simulink model "AC_base_1_VSM_2_22a"  (R2022a)
settings: Solver=ode3  StartTime=0.0  StopTime=8  FixedStep=HWSampleTime  RelTol=1e-3
undefined symbols (not defined in the file): ControlSampleTime, DiscIntNeverNeededParam, HWSampleTime, Ipwm_back, Ipwm_off, LCL, Manage, Oversample, Param, scaling_factor, SM, Ts, V_DC, VSMCTRL
libraries: fl_lib x100, nesl_utility x63, simulink x38, FriedrichLibrary x38, ee_lib x20, simulink_extras x14, TriphaseHardwaremodule x12, spsEdgeDetectorLib x2, StateMachines x2, slpidlib x2, spsPower3phInstantaneousLib x1
(part 4 of 7)

== system AC_base_1_VSM_2_22a/Variant Subsystem3/VSM/VSM1/VSM/Meas ==
  note: Ucap reference frame
  note: VSM Reference Frame
  MEASIN : Inport
  "CONTROL " : Inport  Port=2
  Bus Creator : BusCreator  Inputs=4
  Bus Creator4 : BusCreator  Inputs=10
  Bus Selector : BusSelector  OutputSignals=meas_i_inverter,meas_u_cap,meas_u_out,meas_i_out,meas_vol_dc
  Bus Selector1 : BusSelector  OutputSignals=connection_state,enabled
  Bus Selector2 : BusSelector  OutputSignals=phi_VSM
  Gain{,1..3} (4 alike) : Gain  Gain=eye(3,NrChannels)  Multiplication=Matrix(K*u)
  InstantPowerPhN : FriedrichLibrary/Transformations/InstantPowerPhN  SystemSampleTime=-1  VariantActivationTime=update diagram  Latency=0  AutoFrameSizeCalculation=off
  "InstantPowerPhN " : FriedrichLibrary/Transformations/InstantPowerPhN  SystemSampleTime=-1  VariantActivationTime=update diagram  Latency=0  AutoFrameSizeCalculation=off
  PowerPu : Gain  Gain=2/3
  "PowerPu " : Gain  Gain=2/3
  "SI -> pu" : Subsystem  mask{PU=PU}
      mask prompts: PU "PU System"
      mask DialogControl ParameterGroupVar Prompt: Per Unit
  Signal Specification : SignalSpecification  Dimensions=1
  Signal Specification1 : SignalSpecification  Dimensions=1
  Signal Specification2 : SignalSpecification  Dimensions=3
  Signal Specification3 : SignalSpecification  Dimensions=1
  Symmetrical PLL : FriedrichLibrary/Discrete Stuff/Symmetrical PLL  Kp_PLL=PLL.kp  Ki_PLL=PLL.ki  Kd_PLL=0  Ts=ControlSampleTime
  f2omega : Gain  Gain=2*pi
  meas_i_inv : Subsystem
  meas_i_out : Subsystem
  meas_u_cap : Subsystem
  meas_u_out : Subsystem
  MEAS : Outport  VectorParamsAs1DForOutWhenUnconnected=off
  wires:
  PowerPu/1 -> Bus Creator4/8  "PQ"
  Gain3/1 -> meas_u_out/1(abc)
  meas_u_out/1(u_out_x) -> Bus Creator4/5  "u_out"
  Bus Selector/3 -> Gain3/1  "<meas_u_out>"
  Bus Creator/1 -> Bus Creator4/7  "PLL"
  Bus Selector/4 -> Gain2/1  "<meas_i_out>"
  Gain2/1 -> meas_i_out/1(abc), "InstantPowerPhN "/2
  meas_u_cap/1(u_cap_x) -> Bus Creator4/4  "u_cap"
  meas_i_inv/1(i_inv_x) -> Bus Creator4/3  "i_inv"
  InstantPowerPhN/1 -> PowerPu/1
  Bus Selector/2 -> Gain1/1  "<meas_u_cap>"
  Gain/1 -> InstantPowerPhN/2, meas_i_inv/1(abc)
  Symmetrical PLL/1 -> Signal Specification2/1  "vdq"
  Symmetrical PLL/3 -> Signal Specification/1  "f"
  Symmetrical PLL/2 -> Signal Specification1/1, meas_i_out/2(phi)  "phi"
  Bus Selector/1 -> Gain/1  "<meas_i_inverter>"
  Bus Selector/5 -> Signal Specification3/1  "<meas_vol_dc>"
  MEASIN/1 -> Bus Selector1/1, "SI -> pu"/1(MeasIn)
  "CONTROL "/1 -> Bus Selector2/1
  Signal Specification/1 -> f2omega/1, Bus Creator/3  "f"
  Signal Specification1/1 -> Bus Creator/2  "phi"
  Signal Specification2/1 -> Bus Creator/1  "vdq"
  f2omega/1 -> Bus Creator/4  "omega"
  "SI -> pu"/1(MeasOut) -> Bus Selector/1
  Signal Specification3/1 -> Bus Creator4/10  "u_dc"
  Bus Creator4/1 -> MEAS/1
  Bus Selector1/1 -> Bus Creator4/1  "<connection_state>"
  Bus Selector1/2 -> Bus Creator4/2  "<enabled>"
  Bus Selector2/1 -> meas_i_inv/2(phi), meas_u_out/2(phi), meas_u_cap/2(phi)  "<phi_VSM>"
  "InstantPowerPhN "/1 -> "PowerPu "/1
  "PowerPu "/1 -> Bus Creator4/9  "PQ_out"
  Gain1/1 -> meas_u_cap/1(abc), "InstantPowerPhN "/1, InstantPowerPhN/1, Symmetrical PLL/1
  meas_i_out/1(i_out_x) -> Bus Creator4/6  "i_out"

== system AC_base_1_VSM_2_22a/Variant Subsystem3/VSM/VSM1/command_center/Error ACK ==
  Toggle : Constant  OutMin=0  OutMax=1
  Out : Outport  VectorParamsAs1DForOutWhenUnconnected=off
  wires:
  Toggle/1 -> Out/1

== system AC_base_1_VSM_2_22a/Variant Subsystem3/VSM/VSM1/command_center/Shortcut1 ==

== system AC_base_1_VSM_2_22a/Variant Subsystem3/VSM/VSM1/command_center/Subsystem ==
  In1 : Inport
  In2 : Inport  Port=2
  Enable : EnablePort
  Constant : Constant  Value=4
  Display : Display
  TRI - WP : StateMachines/TRI - WP  Time_Pre1=0.1  T_Pre0=0.1  T_Connect=0.3  T_Disconnect=0.1  T_Enable=0.3  T_Disable=0.1  Time_Error=0.1  Ts=SM.TsTimer
  Terminator : Terminator
  Unit Delay : UnitDelay  SampleTime=ControlSampleTime  HasFrameUpgradeWarning=on
  Unit Delay1 : UnitDelay  SampleTime=ControlSampleTime  HasFrameUpgradeWarning=on
  precharge : Outport
  cmd_ac : Outport  Port=2
  wires:
  TRI - WP/3 -> cmd_ac/1
  In1/1 -> Unit Delay/1
  TRI - WP/4 -> Terminator/1
  Constant/1 -> TRI - WP/1
  Unit Delay1/1 -> TRI - WP/3
  Unit Delay/1 -> TRI - WP/2
  TRI - WP/1 -> Display/1
  TRI - WP/2 -> precharge/1  "precharge"
  In2/1 -> Unit Delay1/1

== system AC_base_1_VSM_2_22a/Variant Subsystem3/VSM/VSM1/command_center/cmd_VSM ==
  note: Parameter
  Bus Creator1 : BusCreator  Inputs=4
  Bus Creator2 : BusCreator  Inputs=2
  Current Control : Subsystem
  Damping : Subsystem
  Manage : Subsystem
  Virtual Circuit : Subsystem
  Virtual Synchronous Machine : Subsystem
  cmd_ac : Outport  VectorParamsAs1DForOutWhenUnconnected=off
  wires:
  Bus Creator2/1 -> cmd_ac/1
  Virtual Synchronous Machine/1(Virtual Synchronous Machine) -> Bus Creator1/1  "VSM"
  Current Control/1(Current Control) -> Bus Creator1/2  "CC"
  Damping/1(Damping) -> Bus Creator1/3  "Damping"
  Virtual Circuit/1(Virtual Circuit) -> Bus Creator1/4  "VC"
  Manage/1(Manage) -> Bus Creator2/1  "Manage"
  Bus Creator1/1 -> Bus Creator2/2  "Param"

== system AC_base_1_VSM_2_22a/Variant Subsystem3/VSM/VSM1/diagPlot/dq->abs1 ==
  dq : Inport
  Abs : Abs  SaturateOnIntegerOverflow=off
  Demux : Demux  Outputs=2
  Real-Imag to Complex : RealImagToComplex
  abs : Outport  VectorParamsAs1DForOutWhenUnconnected=off
  wires:
  Abs/1 -> abs/1
  Demux/2 -> Real-Imag to Complex/2
  dq/1 -> Demux/1
  Real-Imag to Complex/1 -> Abs/1
  Demux/1 -> Real-Imag to Complex/1

== system AC_base_1_VSM_2_22a/Variant Subsystem3/VSM/VSM1/diagPlot/dq0->abs ==
  dq0 : Inport
  Abs : Abs  SaturateOnIntegerOverflow=off
  Demux : Demux  Outputs=3
  Real-Imag to Complex : RealImagToComplex
  Terminator : Terminator
  abs : Outport  VectorParamsAs1DForOutWhenUnconnected=off
  wires:
  Demux/3 -> Terminator/1
  Demux/1 -> Real-Imag to Complex/1
  Real-Imag to Complex/1 -> Abs/1
  dq0/1 -> Demux/1
  Demux/2 -> Real-Imag to Complex/2
  Abs/1 -> abs/1

== system AC_base_1_VSM_2_22a/Variant Subsystem3/VSM/VSM1/diagPlot/dq0->abs2 ==
  dq0 : Inport
  Abs : Abs  SaturateOnIntegerOverflow=off
  Demux : Demux  Outputs=3
  Real-Imag to Complex : RealImagToComplex
  Terminator : Terminator
  abs : Outport  VectorParamsAs1DForOutWhenUnconnected=off
  wires:
  Demux/3 -> Terminator/1
  Demux/1 -> Real-Imag to Complex/1
  Real-Imag to Complex/1 -> Abs/1
  dq0/1 -> Demux/1
  Demux/2 -> Real-Imag to Complex/2
  Abs/1 -> abs/1

== system AC_base_1_VSM_2_22a/Variant Subsystem1/VSM/Inverter AverageMdl LC SimScape2/Modul F30 fixed DC voltage Average SimScape/measMerge3/measMerge123 ==
  note: In Triphase Modell: Mittelwert aus allen dc Spannungen.
      | Da im Modell die DC Spannung identisch ist, wird die erste übergeben
  meas1 : Inport
  meas2 : Inport  Port=2
  meas3 : Inport  Port=3
  Bus Creator : BusCreator  Inputs=3
  Bus Creator2 : BusCreator  Inputs=8
  Bus Selector : BusSelector  OutputSignals=meas1.meas_u_cap,meas2.meas_u_cap,meas3.meas_u_cap
  Bus Selector1 : BusSelector  OutputSignals=meas1.meas_u_out,meas2.meas_u_out,meas3.meas_u_out
  Bus Selector2 : BusSelector  OutputSignals=meas1.meas_i_inverter,meas2.meas_i_inverter,meas3.meas_i_inverter
  Bus Selector3 : BusSelector  OutputSignals=meas1.meas_i_out,meas2.meas_i_out,meas3.meas_i_out
  Bus Selector4 : BusSelector  OutputSignals=meas1.connection_state  OutputAsBus=on
  Bus Selector5 : BusSelector  OutputSignals=meas1.enabled  OutputAsBus=on
  Bus Selector6 : BusSelector  OutputSignals=meas1.meas_u_dc  OutputAsBus=on
  Bus Selector7 : BusSelector  OutputSignals=meas1.block,meas3.block,meas2.block
  Bus to Vector4 : BusToVector  Commented=on
  Mux{,1..4} (5 alike) : Mux  Inputs=3
  meas : Outport  VectorParamsAs1DForOutWhenUnconnected=off
  wires:
  Mux4/1 -> Bus Creator2/8  "block"
  Bus Selector7/3 -> Mux4/3  "<block>"
  Bus Selector7/1 -> Mux4/1  "<block>"
  Bus Selector7/2 -> Mux4/2  "<block>"
  Bus Selector3/3 -> Mux3/3  "<meas_i_out>"
  Bus Selector3/2 -> Mux3/2  "<meas_i_out>"
  Bus Selector3/1 -> Mux3/1  "<meas_i_out>"
  Bus Selector2/3 -> Mux2/3  "<meas_i_inverter>"
  Bus Selector2/2 -> Mux2/2  "<meas_i_inverter>"
  Bus Selector2/1 -> Mux2/1  "<meas_i_inverter>"
  Bus Selector1/3 -> Mux1/3  "<meas_u_out>"
  Bus Selector1/2 -> Mux1/2  "<meas_u_out>"
  Bus Selector1/1 -> Mux1/1  "<meas_u_out>"
  Bus Selector/3 -> Mux/3  "<meas_u_cap>"
  Bus Selector/2 -> Mux/2  "<meas_u_cap>"
  Bus Selector/1 -> Mux/1  "<meas_u_cap>"
  Bus Selector6/1 -> Bus Creator2/1  "meas_u_dc"
  Bus Selector5/1 -> Bus Creator2/7  "enabled"
  Bus Creator/1 -> Bus Selector6/1, Bus Selector/1, Bus Selector1/1, Bus Selector2/1, Bus Selector3/1, Bus Selector4/1, Bus Selector5/1, Bus Selector7/1
  meas2/1 -> Bus Creator/2  "meas2"
  meas1/1 -> Bus Creator/1  "meas1"
  Mux/1 -> Bus Creator2/2  "meas_u_cap"
  Mux1/1 -> Bus Creator2/3  "meas_u_out"
  Mux2/1 -> Bus Creator2/4  "meas_i_inverter"
  Mux3/1 -> Bus Creator2/5  "meas_i_out"
  Bus Creator2/1 -> meas/1
  Bus Selector4/1 -> Bus Creator2/6  "connection_state"
  meas3/1 -> Bus Creator/3  "meas3"

== system AC_base_1_VSM_2_22a/Variant Subsystem1/VSM/Inverter AverageMdl LC SimScape2/Modul F30 fixed DC voltage Average SimScape/simscape_bridgefilter_aca/PWM Blocking1 ==
  i_inverter : Inport
  enable : Inport  Port=2
  AND2 : Logic  IconShape=distinctive  AllPortsSameDT=off  OutDataTypeStr=boolean
  AND3 : Logic  IconShape=distinctive  AllPortsSameDT=off  OutDataTypeStr=boolean
  Abs2 : Abs  SaturateOnIntegerOverflow=off
  Compare To Constant1 : simulink/Logic and Bit Operations/Compare To Constant  relop=<=  const=Ipwm_back  OutDataTypeStr=boolean
  Compare To Constant4 : simulink/Logic and Bit Operations/Compare To Constant  relop=>  const=Ipwm_off  OutDataTypeStr=boolean
  Data Type Conversion2 : DataTypeConversion  SaturateOnIntegerOverflow=off  RndMeth=Floor
  S-R Flip-Flop1 : simulink_extras/Flip Flops/S-R Flip-Flop  initial_condition=0
  Terminator1 : Terminator
  Trigger Spike at new Control Sample : Subsystem
  Unit Delay2 : UnitDelay  SampleTime=-1  HasFrameUpgradeWarning=on
  enable_blk : Outport
  wires:
  i_inverter/1 -> Unit Delay2/1
  S-R Flip-Flop1/2 -> Terminator1/1
  AND3/1 -> Data Type Conversion2/1
  enable/1 -> AND3/1
  Data Type Conversion2/1 -> enable_blk/1
  S-R Flip-Flop1/1 -> AND3/2  "ena"
  Compare To Constant4/1 -> S-R Flip-Flop1/2  "R"
  AND2/1 -> S-R Flip-Flop1/1
  Abs2/1 -> Compare To Constant1/1, Compare To Constant4/1
  Unit Delay2/1 -> Abs2/1
  Compare To Constant1/1 -> AND2/2  "S"
  Trigger Spike at new Control Sample/1(y) -> AND2/1

== system AC_base_1_VSM_2_22a/Variant Subsystem1/VSM/Inverter AverageMdl LC SimScape2/Modul F30 fixed DC voltage Average SimScape/simscape_bridgefilter_aca1/PWM Blocking1 ==
  i_inverter : Inport
  enable : Inport  Port=2
  AND2 : Logic  IconShape=distinctive  AllPortsSameDT=off  OutDataTypeStr=boolean
  AND3 : Logic  IconShape=distinctive  AllPortsSameDT=off  OutDataTypeStr=boolean
  Abs2 : Abs  SaturateOnIntegerOverflow=off
  Compare To Constant1 : simulink/Logic and Bit Operations/Compare To Constant  relop=<=  const=Ipwm_back  OutDataTypeStr=boolean
  Compare To Constant4 : simulink/Logic and Bit Operations/Compare To Constant  relop=>  const=Ipwm_off  OutDataTypeStr=boolean
  Data Type Conversion2 : DataTypeConversion  SaturateOnIntegerOverflow=off  RndMeth=Floor
  S-R Flip-Flop1 : simulink_extras/Flip Flops/S-R Flip-Flop  initial_condition=0
  Terminator1 : Terminator
  Trigger Spike at new Control Sample : Subsystem
  Unit Delay2 : UnitDelay  SampleTime=-1  HasFrameUpgradeWarning=on
  enable_blk : Outport
  wires:
  Trigger Spike at new Control Sample/1(y) -> AND2/1
  Compare To Constant1/1 -> AND2/2  "S"
  Unit Delay2/1 -> Abs2/1
  Abs2/1 -> Compare To Constant4/1, Compare To Constant1/1
  AND2/1 -> S-R Flip-Flop1/1
  Compare To Constant4/1 -> S-R Flip-Flop1/2  "R"
  S-R Flip-Flop1/1 -> AND3/2  "ena"
  Data Type Conversion2/1 -> enable_blk/1
  enable/1 -> AND3/1
  AND3/1 -> Data Type Conversion2/1
  S-R Flip-Flop1/2 -> Terminator1/1
  i_inverter/1 -> Unit Delay2/1

== system AC_base_1_VSM_2_22a/Variant Subsystem1/VSM/Inverter AverageMdl LC SimScape2/Modul F30 fixed DC voltage Average SimScape/simscape_bridgefilter_aca2/PWM Blocking1 ==
  i_inverter : Inport
  enable : Inport  Port=2
  AND2 : Logic  IconShape=distinctive  AllPortsSameDT=off  OutDataTypeStr=boolean
  AND3 : Logic  IconShape=distinctive  AllPortsSameDT=off  OutDataTypeStr=boolean
  Abs2 : Abs  SaturateOnIntegerOverflow=off
  Compare To Constant1 : simulink/Logic and Bit Operations/Compare To Constant  relop=<=  const=Ipwm_back  OutDataTypeStr=boolean
  Compare To Constant4 : simulink/Logic and Bit Operations/Compare To Constant  relop=>  const=Ipwm_off  OutDataTypeStr=boolean
  Data Type Conversion2 : DataTypeConversion  SaturateOnIntegerOverflow=off  RndMeth=Floor
  S-R Flip-Flop1 : simulink_extras/Flip Flops/S-R Flip-Flop  initial_condition=0
  Terminator1 : Terminator
  Trigger Spike at new Control Sample : Subsystem
  Unit Delay2 : UnitDelay  SampleTime=-1  HasFrameUpgradeWarning=on
  enable_blk : Outport
  wires:
  i_inverter/1 -> Unit Delay2/1
  S-R Flip-Flop1/2 -> Terminator1/1
  AND3/1 -> Data Type Conversion2/1
  enable/1 -> AND3/1
  Data Type Conversion2/1 -> enable_blk/1
  S-R Flip-Flop1/1 -> AND3/2  "ena"
  Compare To Constant4/1 -> S-R Flip-Flop1/2  "R"
  AND2/1 -> S-R Flip-Flop1/1
  Abs2/1 -> Compare To Constant1/1, Compare To Constant4/1
  Unit Delay2/1 -> Abs2/1
  Compare To Constant1/1 -> AND2/2  "S"
  Trigger Spike at new Control Sample/1(y) -> AND2/1

== system AC_base_1_VSM_2_22a/Variant Subsystem1/VSM/VSM1/VSM/CONTROL/Subsystem1 ==
  <R1> : Inport
  <L1> : Inport  Port=2
  I : Inport  Port=3
  U_i : Inport  Port=4
  Enable : EnablePort
  MATLAB Function : MATLAB Function  TreatAsAtomicUnit=on  SystemSampleTime=ControlSampleTime
  Selector : Selector  InputPortWidth=3  IndexOptions=Index vector (dialog)  Indices=[1 2]  OutputSizes=1
  Selector1 : Selector  InputPortWidth=3  IndexOptions=Index vector (dialog)  Indices=[1 2]  OutputSizes=1
  phi_vsm : Outport
  U_v : Outport  Port=2
  wires:
  <L1>/1 -> MATLAB Function/2(L1)
  <R1>/1 -> MATLAB Function/3(R1)
  Selector/1 -> MATLAB Function/1(I)
  Selector1/1 -> MATLAB Function/4(U_i)
  I/1 -> Selector/1
  U_i/1 -> Selector1/1
  MATLAB Function/1(phi_vsm) -> phi_vsm/1
  MATLAB Function/2(U_v) -> U_v/1

== system AC_base_1_VSM_2_22a/Variant Subsystem1/VSM/VSM1/VSM/CONTROL/VSMOC1 ==
  Manage : Inport
  Meas : Inport  Port=2
  u_inv_dq : Inport  Port=3
  Bus Selector1 : BusSelector  OutputSignals=enable_VSM.enable_ctrl,Param.VSM,enable_VSM.enable_inertia,sp_VSM
  Bus Selector11 : BusSelector  OutputSignals=phi
  Bus Selector2 : BusSelector  OutputSignals=PQ,PLL,u_cap.u_cap_dq0
  Selector : Selector  InputPortWidth=3  IndexOptions=Index vector (dialog)  Indices=[1 2]  OutputSizes=1
  Switch : Switch  Criteria=u2 ~= 0  SaturateOnIntegerOverflow=off  InputSameDT=off
  VSMOC : Subsystem
  phi_rad : Outport  VectorParamsAs1DForOutWhenUnconnected=off
  sp_u_inv_dq : Outport  Port=2  InitialOutput=[1 0]  VectorParamsAs1DForOutWhenUnconnected=off
  VSMdiag : Outport  Port=3  VectorParamsAs1DForOutWhenUnconnected=off
  wires:
  Bus Selector2/1 -> VSMOC/4(PQ_meas)  "<PQ>"
  Selector/1 -> VSMOC/7(u_cap_dq1)
  Bus Selector2/3 -> Selector/1  "<u_cap_dq0>"
  u_inv_dq/1 -> VSMOC/6(u_inv_dq)
  Bus Selector1/4 -> VSMOC/3(sp_VSM)  "<sp_VSM>"
  Bus Selector1/3 -> VSMOC/2(enable_inertia)  "<enable_inertia>"
  Bus Selector1/2 -> VSMOC/1(Param)  "<VSM>"
  Bus Selector2/2 -> Bus Selector11/1, VSMOC/5(PLL)  "<PLL>"
  Meas/1 -> Bus Selector2/1
  Bus Selector1/1 -> Switch/2, VSMOC/Enable  "<enable_ctrl>"
  Manage/1 -> Bus Selector1/1
  Switch/1 -> phi_rad/1
  VSMOC/2(sp_u_inv_dq) -> sp_u_inv_dq/1
  VSMOC/3(VSMdiag) -> VSMdiag/1
  VSMOC/1(phi_rad) -> Switch/1
  Bus Selector11/1 -> Switch/3  "<phi>"

== system AC_base_1_VSM_2_22a/Variant Subsystem1/VSM/VSM1/VSM/CONTROL/Virtual Circuit mit R und L ==
  Param : Inport
  Reset : Inport  Port=2
  i_dq0 : Inport  Port=3
  Phi : Inport  Port=4
  Bus Selector : BusSelector  OutputSignals=R1,L1
  Bus Selector1 : BusSelector  OutputSignals=R1t,tauR,L1t,tauL
  Current Predictor : Subsystem  Commented=on
  L_Matrix : Gain  Gain=[0 -1 0;1 0 0; 0 0 0]
  L_Matrix1 : Gain  Gain=[0 -1 0;1 0 0; 0 0 0]
  PT1 : Subsystem  mask{K=1, Init=0, Ts=ControlSampleTime}
      mask prompts: K "Gain"; Init "Initial input"; Ts "Sample time"
      mask DialogControl DescGroupVar Prompt: PT1 discrete
      mask DialogControl DescTextVar Prompt: Simple discrete PT1
      mask Display:
      | text(0.5,0.5,get_param(gcb,'K'),'HorizontalAlignment','center','VerticalAlignment','Bottom')
      | text(0.5,0.5,'1 + s.tau','HorizontalAlignment','center','VerticalAlignment','Top')
      | plot([0.3 0.7],[0.5 0.5])
  PT2 : Subsystem  mask{K=1, Init=0, Ts=ControlSampleTime}
      mask prompts: K "Gain"; Init "Initial input"; Ts "Sample time"
      mask DialogControl DescGroupVar Prompt: PT1 discrete
      mask DialogControl DescTextVar Prompt: Simple discrete PT1
      mask Display:
      | text(0.5,0.5,get_param(gcb,'K'),'HorizontalAlignment','center','VerticalAlignment','Bottom')
      | text(0.5,0.5,'1 + s.tau','HorizontalAlignment','center','VerticalAlignment','Top')
      | plot([0.3 0.7],[0.5 0.5])
  "Param " : InportShadow
  Phi1 : InportShadow  Port=4
  Product : Product  Multiplication=Matrix(*)
  Product1 : Product  Multiplication=Matrix(*)
  Product2 : Product  Multiplication=Matrix(*)
  R_Matrix : Gain  Gain=[1 0 0;0 1 0; 0 0 0]
  R_Matrix1 : Gain  Gain=[1 0 0;0 1 0; 0 0 0]
  Reset1 : InportShadow  Port=2
  Sum : Sum  Inputs=++|
  Sum1 : Sum  Inputs=++|
  Sum2 : Sum  Inputs=|++
  " u_dq0" : Outport
  wires:
  Product/1 -> Sum2/1
  PT2/1(Y) -> Product2/2
  Reset1/1 -> PT2/3(Reset)
  Reset/1 -> PT1/3(Reset)
  Phi1/1 -> PT2/4(Phi)
  Phi/1 -> PT1/4(Phi)
  PT1/1(Y) -> Product1/2
  Sum2/1 -> " u_dq0"/1
  Product2/1 -> Sum1/2
  L_Matrix1/1 -> Product2/1
  Bus Selector1/3 -> L_Matrix1/1  "<L1t>"
  Bus Selector1/2 -> PT1/2(tau)  "<tauR>"
  Bus Selector1/4 -> PT2/2(tau)  "<tauL>"
  Bus Selector1/1 -> R_Matrix1/1  "<R1t>"
  Product1/1 -> Sum1/1
  R_Matrix1/1 -> Product1/1
  "Param "/1 -> Bus Selector1/1
  Sum/1 -> Product/1
  R_Matrix/1 -> Sum/2
  L_Matrix/1 -> Sum/1
  Bus Selector/2 -> L_Matrix/1  "<L1>"
  i_dq0/1 -> PT1/1(U), PT2/1(U), Product/2
  Bus Selector/1 -> R_Matrix/1  "<R1>"
  Param/1 -> Bus Selector/1

== system AC_base_1_VSM_2_22a/Variant Subsystem1/VSM/VSM1/VSM/CONTROL/Virtual Circuit1 ==
  Param : Inport
  Reset : Inport  Port=2
  i_dq0 : Inport  Port=3
  Phi : Inport  Port=4
  Bus Selector : BusSelector  OutputSignals=R1,L1
  Bus Selector1 : BusSelector  OutputSignals=R1t,tauR,L1t,tauL
  Current Predictor : Subsystem  Commented=on
  L_Matrix : Gain  Gain=[0 -1 0;1 0 0; 0 0 0]
  L_Matrix1 : Gain  Gain=[0 -1 0;1 0 0; 0 0 0]
  PT1 : Subsystem  mask{K=1, Init=0, Ts=ControlSampleTime}
      mask prompts: K "Gain"; Init "Initial input"; Ts "Sample time"
      mask DialogControl DescGroupVar Prompt: PT1 discrete
      mask DialogControl DescTextVar Prompt: Simple discrete PT1
      mask Display:
      | text(0.5,0.5,get_param(gcb,'K'),'HorizontalAlignment','center','VerticalAlignment','Bottom')
      | text(0.5,0.5,'1 + s.tau','HorizontalAlignment','center','VerticalAlignment','Top')
      | plot([0.3 0.7],[0.5 0.5])
  PT2 : Subsystem  Commented=on  mask{K=1, Init=0, Ts=ControlSampleTime}
      mask prompts: K "Gain"; Init "Initial input"; Ts "Sample time"
      mask DialogControl DescGroupVar Prompt: PT1 discrete
      mask DialogControl DescTextVar Prompt: Simple discrete PT1
      mask Display:
      | text(0.5,0.5,get_param(gcb,'K'),'HorizontalAlignment','center','VerticalAlignment','Bottom')
      | text(0.5,0.5,'1 + s.tau','HorizontalAlignment','center','VerticalAlignment','Top')
      | plot([0.3 0.7],[0.5 0.5])
  "Param " : InportShadow
  Phi1 : InportShadow  Port=4
  Product : Product  Multiplication=Matrix(*)
  Product1 : Product  Multiplication=Matrix(*)
  Product2 : Product  Commented=on  Multiplication=Matrix(*)
  Product3 : Product  Multiplication=Matrix(*)
  R_Matrix : Gain  Gain=[1 0 0;0 1 0; 0 0 0]
  R_Matrix1 : Gain  Gain=[1 0 0;0 1 0; 0 0 0]
  Reset1 : InportShadow  Port=2
  Scope : Scope  NumInputPorts=2
  Scope1 : Scope
  Sum : Sum  Inputs=++|
  Sum1 : Sum  Inputs=++|
  Sum2 : Sum  Inputs=|++
  " u_dq0" : Outport
  wires:
  Product3/1 -> Scope/1
  Reset1/1 -> PT2/3(Reset)
  Reset/1 -> PT1/3(Reset)
  Phi1/1 -> PT2/4(Phi)
  PT1/1(Y) -> Product1/2
  Sum2/1 -> " u_dq0"/1
  Sum1/1 -> Sum2/2
  Product2/1 -> Sum1/2, Scope1/1
  PT2/1(Y) -> Product2/2
  L_Matrix1/1 -> Product2/1
  Bus Selector1/3 -> L_Matrix1/1  "<L1t>"
  Bus Selector1/2 -> PT1/2(tau)  "<tauR>"
  Bus Selector1/4 -> PT2/2(tau)  "<tauL>"
  Bus Selector1/1 -> R_Matrix1/1  "<R1t>"
  Product1/1 -> Sum1/1, Scope/2
  R_Matrix1/1 -> Product1/1
  Product/1 -> Sum2/1
  "Param "/1 -> Bus Selector1/1
  Sum/1 -> Product/1
  R_Matrix/1 -> Sum/2, Product3/1
  L_Matrix/1 -> Sum/1
  Bus Selector/2 -> L_Matrix/1  "<L1>"
  i_dq0/1 -> Product/2, Product3/2, PT1/1(U), PT2/1(U)
  Bus Selector/1 -> R_Matrix/1  "<R1>"
  Param/1 -> Bus Selector/1

== system AC_base_1_VSM_2_22a/Variant Subsystem1/VSM/VSM1/VSM/CONTROL/active_damping ==
  enable_damp_dq : Inport
  Reset : Inport  Port=2
  u_dq0 : Inport  Port=3
  Phi : Inport  Port=4
  Bus Selector : BusSelector  OutputSignals=Damp_dq,Damp_dq,Damp_CM,OmLead,OmLag
  Integrator (inertia) : DiscreteIntegrator  gainval=1  ExternalReset=rising  InitialConditionSource=external  InitialCondition=1  SampleTime=ControlSampleTime  ICPrevOutput=DiscIntNeverNeededParam  ICPrevScaledInput=DiscIntNeverNeededParam
  Mux : Mux  Inputs=3
  Product{,1..3} (4 alike) : Product
  Sum : Sum  Inputs=|+-
  Sum2 : Sum  Inputs=++|
  Unit Delay2 : UnitDelay  InitialCondition=[0 0 0]  SampleTime=ControlSampleTime  HasFrameUpgradeWarning=on
  dq0->ab0 phi : FriedrichLibrary/Transformations/dq0->ab0 phi  SystemSampleTime=-1  VariantActivationTime=update diagram  Latency=0  AutoFrameSizeCalculation=off
  damp_dq0 : Outport  VectorParamsAs1DForOutWhenUnconnected=off
  wires:
  Bus Selector/5 -> Product3/2  "<OmLag>"
  Bus Selector/4 -> Product2/1  "<OmLead>"
  dq0->ab0 phi/1 -> Integrator (inertia)/3
  Unit Delay2/1 -> dq0->ab0 phi/1
  Reset/1 -> Integrator (inertia)/2
  Phi/1 -> dq0->ab0 phi/2
  Product1/1 -> damp_dq0/1
  Mux/1 -> Product/1, Product1/1  "enable"
  Product/1 -> Product2/2, Sum2/1
  u_dq0/1 -> Product/2
  Bus Selector/3 -> Mux/3  "<Damp_CM>"
  Bus Selector/2 -> Mux/2  "<Damp_dq>"
  Bus Selector/1 -> Mux/1  "<Damp_dq>"
  enable_damp_dq/1 -> Bus Selector/1
  Sum/1 -> Integrator (inertia)/1
  Sum2/1 -> Product1/2, Product3/1
  Product3/1 -> Sum/2
  Integrator (inertia)/1 -> Sum2/2, Unit Delay2/1
  Product2/1 -> Sum/1

== system AC_base_1_VSM_2_22a/Variant Subsystem1/VSM/VSM1/VSM/CONTROL/dq0 to duty ==
  phi_rad : Inport
  u_dq0 : Inport  Port=2
  u_dc : Inport  Port=3
  Bias : Bias  Bias=Ctrl.PWM.tauT*Ctrl.PU.omegab  SaturateOnIntegerOverflow=off
  Bus Creator3 : BusCreator  Inputs=2
  Divide : Product  Inputs=*/
  Gain : Gain  Gain=eye(NrChannels,3)  Multiplication=Matrix(K*u)
  Modulation : FriedrichLibrary/Transformations/Modulation  Method=Sine Modulation  Ts=ControlSampleTime
  SMA : FriedrichLibrary/Discrete Stuff/SMA  n_samples=1/ControlSampleTime/100  init_out=0
  Saturation : Saturate  UpperLimit=inf  LowerLimit=1
  Signal Specification1 : SignalSpecification
  dq0->ab0 phi : FriedrichLibrary/Transformations/dq0->ab0 phi  SystemSampleTime=-1  VariantActivationTime=update diagram  Latency=0  AutoFrameSizeCalculation=off
  d : Outport  VectorParamsAs1DForOutWhenUnconnected=off
  pwmDiag : Outport  Port=2  VectorParamsAs1DForOutWhenUnconnected=off
  wires:
  SMA/1 -> Divide/2
  Saturation/1 -> SMA/1
  Signal Specification1/1 -> d/1
  Gain/1 -> Signal Specification1/1, Bus Creator3/1  "pwm"
  Bus Creator3/1 -> pwmDiag/1  "pwmDiag"
  u_dc/1 -> Saturation/1
  Bias/1 -> dq0->ab0 phi/2
  Modulation/1 -> Gain/1
  dq0->ab0 phi/1 -> Divide/1
  Divide/1 -> Modulation/1  "ab0 norm"
  u_dq0/1 -> dq0->ab0 phi/1
  phi_rad/1 -> Bias/1, Bus Creator3/2  "phi"

== system AC_base_1_VSM_2_22a/Variant Subsystem1/VSM/VSM1/VSM/CONTROL/i_dq_ctrl ==
  note: PI Control
  note: Outrouting
  note: Inrouting
  Param : Inport
  enable_cc : Inport  Port=2
  sp_cc : Inport  Port=3
  ms_i_inv_dq : Inport  Port=4
  u_ff_dq : Inport  Port=5
  u_inv_dq : Inport  Port=6
  Enable : EnablePort  StatesWhenEnabling=reset
  Bus Creator2 : BusCreator  Inputs=4
  Bus Selector13 : BusSelector  OutputSignals=init_u_inv
  Constant : Constant
  Demux : Demux  Outputs=2
  From1 : From  Commented=on  GotoTag=initU
  Gain1 : Gain  Commented=on  Gain=Kff
  Gain2 : Gain  Gain=L_inv
  Gain4 : Gain  Gain=[0 -1;1 0]  Multiplication=Matrix(K*u)
  Gain5 : Gain  Commented=on  Gain=1-Kff
  Mux : Mux  Inputs=2
  PI : Subsystem
  Product : Product
  Product1 : Product
  Product2 : Product
  Scope : Scope  NumInputPorts=3
  Step : Step  Time=8  Before=1  After=0  SampleTime=0
  Sum1 : Sum  Inputs=+++
  Sum2 : Sum  Commented=on  Inputs=|+-
  Sum3 : Sum  Inputs=|+-
  Switch1 : Switch  Commented=on  Criteria=u2 > Threshold  SaturateOnIntegerOverflow=off  InputSameDT=off
  sp_u_inv_dq : Outport  VectorParamsAs1DForOutWhenUnconnected=off
  CCdiag : Outport  Port=2  VectorParamsAs1DForOutWhenUnconnected=off
  wires:
  PI/1(u) -> Sum1/1  "pi"
  Constant/1 -> Product1/2, Product2/2
  Demux/1 -> Product2/1
  Product2/1 -> Mux/1
  Product1/1 -> Mux/2
  Demux/2 -> Product1/1
  Mux/1 -> PI/1(di)
  ms_i_inv_dq/1 -> Gain4/1, Sum3/2, [i_dq]
  Product/1 -> [sp_u_dq], sp_u_inv_dq/1
  Gain5/1 -> Switch1/3
  u_ff_dq/1 -> Gain5/1, Gain1/1, PI/2(u0), Scope/2
  [i_dq] -> Bus Creator2/2  "i_dq"
  [sp_i_dq] -> Bus Creator2/1  "sp_i_dq"
  Bus Creator2/1 -> CCdiag/1
  [Enable] -> Bus Creator2/4  "enable_cc"
  enable_cc/1 -> [Enable]  "enable_cc"
  [sp_u_dq] -> Bus Creator2/3  "sp_u_dq"
  [Enable] -> Product/1
  Bus Selector13/1 -> [initU]  "<init_u_inv>"
  Param/1 -> Bus Selector13/1
  sp_cc/1 -> Sum3/1, [sp_i_dq]
  Sum3/1 -> Demux/1
  [Enable] -> PI/Enable
  u_inv_dq/1 -> Switch1/1
  Sum1/1 -> Product/2, Scope/1
  From1/1 -> Switch1/2
  Gain2/1 -> Sum2/2  "dq decouple"
  Gain4/1 -> Gain2/1
  Switch1/1 -> Sum2/1

== system AC_base_1_VSM_2_22a/Variant Subsystem1/VSM/VSM1/VSM/MANAGEMENT/Subsystem1 ==
  i_inv_ab : Inport
  <i_inv_dq0> : Inport  Port=2
  <u_cap_ab0> : Inport  Port=3
  <PQ_out> : Inport  Port=4
  enable : Inport  Port=5
  i_out_ab : Inport  Port=6
  "AL brechen AL nicht mit FCN lösbar " : Memory
  Compare To Constant : simulink/Logic and Bit Operations/Compare To Constant  relop===  const=0  OutDataTypeStr=boolean
  Complex to Magnitude-Angle : ComplexToMagnitudeAngle
  Demux : Demux  Outputs=2
  Divide : Product  Inputs=*/
  Enabled Subsystem : Subsystem  TreatAsAtomicUnit=on
  Math Function1 : Math  Operator=square  SignedPower=on
  Math Function2 : Math  Operator=square  SignedPower=on
  Math Function3 : Math  Operator=square  SignedPower=on
  Max : MinMax  Function=max  Inputs=2
  Real-Imag to Complex : RealImagToComplex
  Scope : Scope  NumInputPorts=2
  Selector2 : Selector  InputPortWidth=3  IndexOptions=Index vector (dialog)  Indices=[1 2]  OutputSizes=1
  Sqrt1 : Sqrt
  Sqrt2 : Sqrt
  Sqrt3 : Sqrt
  Subsystem : Subsystem
  Sum of Elements1 : Sum  Inputs=+
  Sum of Elements2 : Sum  Inputs=+
  Sum of Elements3 : Sum  Inputs=+
  Transport Delay : TransportDelay  DelayTime=0.1
  Transport Delay1 : TransportDelay  DelayTime=0.1
  Unit Delay : UnitDelay  SampleTime=ControlSampleTime  HasFrameUpgradeWarning=on
  Unit Delay1 : UnitDelay  SampleTime=ControlSampleTime  HasFrameUpgradeWarning=on
  CC : Outport
  sp_CC : Outport  Port=2
  wires:
  Complex to Magnitude-Angle/2 -> Subsystem/7(angle_i)
  Real-Imag to Complex/1 -> Complex to Magnitude-Angle/1
  Divide/1 -> Transport Delay1/1, Demux/1
  Demux/2 -> Real-Imag to Complex/2
  Demux/1 -> Real-Imag to Complex/1
  Max/1 -> Subsystem/3(iabs)
  Sqrt2/1 -> Transport Delay/1, Max/2
  Sqrt3/1 -> Max/1
  i_out_ab/1 -> Math Function3/1
  Sum of Elements3/1 -> Sqrt3/1
  Math Function3/1 -> Sum of Elements3/1
  Transport Delay1/1 -> Enabled Subsystem/2(i_pq)
  Unit Delay1/1 -> Subsystem/5(PQ_pre)
  Enabled Subsystem/2(i_pq_pre) -> Scope/2, Unit Delay1/1
  Unit Delay/1 -> Subsystem/6(i abs_pre)
  Transport Delay/1 -> Enabled Subsystem/1(i_abs)
  Subsystem/3(set) -> Compare To Constant/1
  Enabled Subsystem/1(i abs_pre) -> Unit Delay/1, Scope/1
  Compare To Constant/1 -> Enabled Subsystem/Enable
  enable/1 -> Subsystem/Enable
  <PQ_out>/1 -> Subsystem/2(PQ_out), Divide/1
  Subsystem/2(CC) -> CC/1
  i_inv_ab/1 -> Math Function1/1
  Subsystem/1(i_sp) -> sp_CC/1  "sp_CC"
  <i_inv_dq0>/1 -> "AL brechen AL nicht mit FCN lösbar "/1
  <u_cap_ab0>/1 -> Selector2/1
  Math Function2/1 -> Sum of Elements2/1
  Sqrt1/1 -> Divide/2, Subsystem/4(U_cap)
  "AL brechen AL nicht mit FCN lösbar "/1 -> Subsystem/1(i_inv)
  Sum of Elements2/1 -> Sqrt1/1
  Math Function1/1 -> Sum of Elements1/1
  Selector2/1 -> Math Function2/1
  Sum of Elements1/1 -> Sqrt2/1

== system AC_base_1_VSM_2_22a/Variant Subsystem1/VSM/VSM1/VSM/MANAGEMENT/current_watchdog ==
  |i| set : Inport
  |i| reset : Inport  Port=2
  i_ab : Inport  Port=3
  sp_gain : Inport  Port=4
  PQ : Inport  Port=5
  i_inv : Inport  Port=6
  active_current_watchdog : EnablePort  StatesWhenEnabling=reset
  Divide : Product  Inputs=/**
  MATLAB Function : MATLAB Function  Commented=on  TreatAsAtomicUnit=on
  Math Function1 : Math  Operator=square  SignedPower=on
  Math Function2 : Math  Operator=square  SignedPower=on
  Math Function3 : Math  Operator=square  SignedPower=on
  Relational Operator : RelationalOperator  Operator=<=  OutDataTypeStr=boolean  InputSameDT=off
  Relational Operator1 : RelationalOperator  Operator=<=  OutDataTypeStr=boolean  InputSameDT=off
  S-R Flip-Flop1 : simulink_extras/Flip Flops/S-R Flip-Flop  initial_condition=0
  Scope : Scope  NumInputPorts=3
  Scope1 : Scope
  Sum of Elements1 : Sum  Inputs=+
  Terminator1 : Terminator
  enable_cc : Outport  VectorParamsAs1DForOutWhenUnconnected=off
  sp_gain_wd : Outport  Port=2  VectorParamsAs1DForOutWhenUnconnected=off
  wires:
  i_inv/1 -> MATLAB Function/4(i_inv)
  PQ/1 -> MATLAB Function/3(p), Scope1/1
  MATLAB Function/2(i) -> sp_gain_wd/1
  MATLAB Function/1(CC) -> Scope/1, enable_cc/1
  sp_gain/1 -> Divide/3
  |i| set/1 -> Math Function2/1, Divide/1
  |i| reset/1 -> Math Function3/1, Divide/2
  Math Function3/1 -> Relational Operator1/2
  S-R Flip-Flop1/2 -> Terminator1/1
  Relational Operator1/1 -> S-R Flip-Flop1/2
  Math Function1/1 -> Sum of Elements1/1
  Sum of Elements1/1 -> Relational Operator/2, MATLAB Function/1(abs), Relational Operator1/1
  i_ab/1 -> Math Function1/1
  Math Function2/1 -> MATLAB Function/2(set), Relational Operator/1

== system AC_base_1_VSM_2_22a/Variant Subsystem1/VSM/VSM1/VSM/MANAGEMENT/sp_VSM ==
  EnableRateLimit : Inport
  CMD : Inport  Port=2
  MEAS : Inport  Port=3
  Bus Creator : BusCreator  Inputs=3
  Bus Selector1 : BusSelector  OutputSignals=u_out.u_out_ab0
  Bus Selector6 : BusSelector  OutputSignals=Param.VSM.sp_f,Param.VSM.sp_E,Param.VSM.sp_PQ,Param.VSM.sp_PQ_limit
  "CMD " : InportShadow  Port=2
  E(PQ) : Subsystem
  PQ(U) Limit : Subsystem
  RateLimit : Subsystem
  Saturation : Saturate  UpperLimit=1  LowerLimit=-1
  sp_VSM : Outport  VectorParamsAs1DForOutWhenUnconnected=off
  wires:
  Saturation/1 -> RateLimit/1(PQ)
  "CMD "/1 -> E(PQ)/2(cmd)
  Bus Creator/1 -> sp_VSM/1
  Bus Selector6/1 -> Bus Creator/1  "<sp_f>"
  MEAS/1 -> Bus Selector1/1
  CMD/1 -> Bus Selector6/1
  PQ(U) Limit/1(sp_PQ_limit) -> Bus Creator/3  "sp_PQ"
  Bus Selector6/4 -> PQ(U) Limit/2(enable)  "<sp_PQ_limit>"
  Bus Selector1/1 -> PQ(U) Limit/3(u_out)  "<u_out_ab0>"
  RateLimit/1(PQslow) -> PQ(U) Limit/1(sp_PQ), E(PQ)/3(sp_PQ)
  EnableRateLimit/1 -> RateLimit/Enable  "ENABLED"
  Bus Selector6/3 -> Saturation/1  "<sp_PQ>"
  Bus Selector6/2 -> E(PQ)/1(E)  "<sp_E>"
  E(PQ)/1(sp_E) -> Bus Creator/2  "sp_E"

== system AC_base_1_VSM_2_22a/Variant Subsystem1/VSM/VSM1/VSM/Meas/SI -> pu ==
  MeasIn : Inport
  Bus Creator1 : BusCreator  Inputs=5
  Bus Selector : BusSelector  OutputSignals=meas_u_out,meas_i_out,meas_i_inverter,meas_u_dc,meas_u_cap
  Normalize : Gain  Gain=1/PU.Ub  OutDataTypeStr=double  RndMeth=Round
  Normalize1 : Gain  Gain=1/PU.Ib  OutDataTypeStr=double  RndMeth=Round
  Normalize2 : Gain  Gain=1/PU.Ib  OutDataTypeStr=double  RndMeth=Round
  Normalize3 : Gain  Gain=1/PU.Ub  OutDataTypeStr=double  RndMeth=Round
  Normalize4 : Gain  Gain=1/PU.Ub/2  OutDataTypeStr=double  RndMeth=Round
  MeasOut : Outport  VectorParamsAs1DForOutWhenUnconnected=off
  wires:
  MeasIn/1 -> Bus Selector/1
  Normalize/1 -> Bus Creator1/1  "meas_u_out"
  Normalize1/1 -> Bus Creator1/3  "meas_i_inverter"
  Normalize2/1 -> Bus Creator1/2  "meas_i_out"
  Normalize4/1 -> Bus Creator1/4  "meas_vol_dc"
  Bus Creator1/1 -> MeasOut/1
  Bus Selector/1 -> Normalize/1  "<meas_u_out>"
  Bus Selector/2 -> Normalize2/1  "<meas_i_out>"
  Bus Selector/3 -> Normalize1/1  "<meas_i_inverter>"
  Bus Selector/4 -> Normalize4/1  "<meas_u_dc>"
  Bus Selector/5 -> Normalize3/1  "<meas_u_cap>"
  Normalize3/1 -> Bus Creator1/5  "meas_u_cap"

== system AC_base_1_VSM_2_22a/Variant Subsystem1/VSM/VSM1/VSM/Meas/meas_i_inv ==
  abc : Inport
  phi : Inport  Port=2
  Bus Creator1 : BusCreator  Inputs=3
  PhN->ab2 : FriedrichLibrary/Transformations/PhN->ab0  SystemSampleTime=-1  VariantActivationTime=update diagram  Latency=0  AutoFrameSizeCalculation=off
  ab0->dq0-faster : FriedrichLibrary/Transformations/ab0->dq0-faster  SystemSampleTime=-1  VariantActivationTime=update diagram  Latency=0  AutoFrameSizeCalculation=off
  i_inv_x : Outport  VectorParamsAs1DForOutWhenUnconnected=off
  wires:
  Bus Creator1/1 -> i_inv_x/1
  phi/1 -> ab0->dq0-faster/2
  abc/1 -> PhN->ab2/1, Bus Creator1/1  "i_inv_abc"
  PhN->ab2/1 -> ab0->dq0-faster/1, Bus Creator1/2  "i_inv_ab0"
  ab0->dq0-faster/1 -> Bus Creator1/3  "i_inv_dq0"

== system AC_base_1_VSM_2_22a/Variant Subsystem1/VSM/VSM1/VSM/Meas/meas_i_out ==
  abc : Inport
  phi : Inport  Port=2
  Bus Creator1 : BusCreator  Inputs=3
  PhN->ab2 : FriedrichLibrary/Transformations/PhN->ab0  SystemSampleTime=-1  VariantActivationTime=update diagram  Latency=0  AutoFrameSizeCalculation=off
  ab0->dq0-faster : FriedrichLibrary/Transformations/ab0->dq0-faster  SystemSampleTime=-1  VariantActivationTime=update diagram  Latency=0  AutoFrameSizeCalculation=off
  i_out_x : Outport  VectorParamsAs1DForOutWhenUnconnected=off
  wires:
  Bus Creator1/1 -> i_out_x/1
  phi/1 -> ab0->dq0-faster/2
  abc/1 -> PhN->ab2/1, Bus Creator1/1  "i_out_abc"
  PhN->ab2/1 -> ab0->dq0-faster/1, Bus Creator1/2  "i_out_ab0"
  ab0->dq0-faster/1 -> Bus Creator1/3  "i_out_dq0"

== system AC_base_1_VSM_2_22a/Variant Subsystem1/VSM/VSM1/VSM/Meas/meas_u_cap ==
  abc : Inport
  phi : Inport  Port=2
  Bus Creator1 : BusCreator  Inputs=3
  PhN->ab2 : FriedrichLibrary/Transformations/PhN->ab0  SystemSampleTime=-1  VariantActivationTime=update diagram  Latency=0  AutoFrameSizeCalculation=off
  ab0->dq0-faster : FriedrichLibrary/Transformations/ab0->dq0-faster  SystemSampleTime=-1  VariantActivationTime=update diagram  Latency=0  AutoFrameSizeCalculation=off
  u_cap_x : Outport  VectorParamsAs1DForOutWhenUnconnected=off
  wires:
  ab0->dq0-faster/1 -> Bus Creator1/3  "u_cap_dq0"
  PhN->ab2/1 -> Bus Creator1/2, ab0->dq0-faster/1  "u_cap_ab0"
  abc/1 -> Bus Creator1/1, PhN->ab2/1  "u_cap_abc"
  phi/1 -> ab0->dq0-faster/2
  Bus Creator1/1 -> u_cap_x/1

== system AC_base_1_VSM_2_22a/Variant Subsystem1/VSM/VSM1/VSM/Meas/meas_u_out ==
  abc : Inport
  phi : Inport  Port=2
  Bus Creator1 : BusCreator  Inputs=3
  PhN->ab2 : FriedrichLibrary/Transformations/PhN->ab0  SystemSampleTime=-1  VariantActivationTime=update diagram  Latency=0  AutoFrameSizeCalculation=off
  ab0->dq0-faster : FriedrichLibrary/Transformations/ab0->dq0-faster  SystemSampleTime=-1  VariantActivationTime=update diagram  Latency=0  AutoFrameSizeCalculation=off
  u_out_x : Outport  VectorParamsAs1DForOutWhenUnconnected=off
  wires:
  ab0->dq0-faster/1 -> Bus Creator1/3  "u_out_dq0"
  PhN->ab2/1 -> Bus Creator1/2, ab0->dq0-faster/1  "u_out_ab0"
  abc/1 -> Bus Creator1/1, PhN->ab2/1  "u_out_abc"
  phi/1 -> ab0->dq0-faster/2
  Bus Creator1/1 -> u_out_x/1

== system AC_base_1_VSM_2_22a/Variant Subsystem1/VSM/VSM1/command_center/cmd_VSM/Current Control ==
  note: else: init with u cap
  Bus Creator6 : BusCreator  Inputs=5
  Bus Creator7 : BusCreator  Inputs=3
  Init with u_inv [0/1] : Constant  Value=VSMCTRL.CC.init_uinv
  activate : Constant  Value=VSMCTRL.CC.activate
  external_stop_cc1 : Constant  Value=0
  external_stop_cc4 : Constant  Value=0
  i_reset_abs : Constant  Value=VSMCTRL.CC.i_reset
  i_set_abs : Constant  Value=VSMCTRL.CC.i_set
  i_sp_gain : Constant  Value=VSMCTRL.CC.i_sp_gain
  Current Control : Outport  VectorParamsAs1DForOutWhenUnconnected=off
  wires:
  Bus Creator6/1 -> Current Control/1  "CC"
  Init with u_inv [0/1]/1 -> Bus Creator6/1  "init_u_inv"
  external_stop_cc1/1 -> Bus Creator6/3  "ex_stop_cc"
  i_sp_gain/1 -> Bus Creator6/4  "i_sp_gain"
  i_set_abs/1 -> Bus Creator7/2  "abs_i_set"
  external_stop_cc4/1 -> Bus Creator6/2  "ex_start_cc"
  Bus Creator7/1 -> Bus Creator6/5  "watchdog"
  i_reset_abs/1 -> Bus Creator7/3  "abs_i_reset"
  activate/1 -> Bus Creator7/1  "activate"

== system AC_base_1_VSM_2_22a/Variant Subsystem1/VSM/VSM1/command_center/cmd_VSM/Damping ==
  Bus Creator5 : BusCreator  Inputs=4
  EnableDamp_CM [0/1] : Constant  Value=VSMCTRL.VTFF.EnableCM
  EnableDamp_dq [0/1] : Constant  Value=VSMCTRL.VTFF.EnableDQ
  Omega Lag : Constant  Value=VSMCTRL.VTFF.OmLag
  Omega Lead : Constant  Value=VSMCTRL.VTFF.OmLead
  Damping : Outport  VectorParamsAs1DForOutWhenUnconnected=off
  wires:
  Omega Lag/1 -> Bus Creator5/4  "OmLag"
  Omega Lead/1 -> Bus Creator5/3  "OmLead"
  Bus Creator5/1 -> Damping/1
  EnableDamp_dq [0/1]/1 -> Bus Creator5/1  "Damp_dq"
  EnableDamp_CM [0/1]/1 -> Bus Creator5/2  "Damp_CM"

== system AC_base_1_VSM_2_22a/Variant Subsystem1/VSM/VSM1/command_center/cmd_VSM/Manage ==
  Bus Creator : BusCreator  Inputs=2
  connect : Constant
  enable : Constant
  Manage : Outport  VectorParamsAs1DForOutWhenUnconnected=off
  wires:
  enable/1 -> Bus Creator/2  "enable"
  connect/1 -> Bus Creator/1  "connect"
  Bus Creator/1 -> Manage/1

== system AC_base_1_VSM_2_22a/Variant Subsystem1/VSM/VSM1/command_center/cmd_VSM/Virtual Circuit ==
  Bus Creator9 : BusCreator  Inputs=7
  Virtual L1 : Constant  Value=VSMCTRL.VC.L1
  Virtual L1t : Constant  Value=VSMCTRL.VC.L1t
  Virtual R1 : Constant  Value=VSMCTRL.VC.R1
  Virtual R1t : Constant  Value=VSMCTRL.VC.R1t
  tau HP Slow : Constant  Value=VSMCTRL.VC.tauSlow
  tau Virtual L1 : Constant  Value=VSMCTRL.VC.tauL
  tau Virtual R1 : Constant  Value=VSMCTRL.VC.tauR
  Virtual Circuit : Outport  VectorParamsAs1DForOutWhenUnconnected=off
  wires:
  tau HP Slow/1 -> Bus Creator9/7  "tauS"
  tau Virtual L1/1 -> Bus Creator9/6  "tauL"
  tau Virtual R1/1 -> Bus Creator9/5  "tauR"
  Virtual L1/1 -> Bus Creator9/3  "L1"
  Bus Creator9/1 -> Virtual Circuit/1
  Virtual L1t/1 -> Bus Creator9/4  "L1t"
  Virtual R1t/1 -> Bus Creator9/2  "R1t"
  Virtual R1/1 -> Bus Creator9/1  "R1"

== system AC_base_1_VSM_2_22a/Variant Subsystem1/VSM/VSM1/command_center/cmd_VSM/Virtual Synchronous Machine ==
  note: 0 Dekaktiviert Init Tiefpass
  note: 0 Dekaktiviert Init Tiefpass
  Bus Creator3 : BusCreator  Inputs=12
  E(sp_PQ) : Constant  Value=VSMCTRL.SP.E_comp
  Ta : Constant  Value=VSMCTRL.VSM.Ta
  Ta1 : Constant  Value=VSMCTRL.VSM.kpf
  Ta2 : Constant  Value=VSMCTRL.VSM.kdf
  Ta3 : Constant  Value=VSMCTRL.VSM.ku
  Ta4 : Constant  Value=VSMCTRL.VSM.Tu
  Ta5 : Constant  Value=0
  Ta6 : Constant  Value=0
  sp_E [pu] : Constant  Value=VSMCTRL.SP.E
  sp_PQ [pu] : Constant  Value=VSMCTRL.SP.PQ
  sp_PQ(U) limit : Constant  Value=VSMCTRL.SP.PQU_lim
  sp_f [Hz] : Constant  Value=VSMCTRL.SP.f
  Virtual Synchronous Machine : Outport  VectorParamsAs1DForOutWhenUnconnected=off
  wires:
  E(sp_PQ)/1 -> Bus Creator3/12  "sp_E_comp"
  Ta5/1 -> Bus Creator3/6  "Tuinit"
  Ta6/1 -> Bus Creator3/7  "TPinit"
  Ta1/1 -> Bus Creator3/2  "kpf"
  Ta2/1 -> Bus Creator3/3  "kdf"
  Ta3/1 -> Bus Creator3/4  "ku"
  Ta4/1 -> Bus Creator3/5  "Tu"
  Bus Creator3/1 -> Virtual Synchronous Machine/1
  Ta/1 -> Bus Creator3/1  "Ta"
  sp_PQ(U) limit/1 -> Bus Creator3/11  "sp_PQ_limit"
  sp_f [Hz]/1 -> Bus Creator3/8  "sp_f"
  sp_PQ [pu]/1 -> Bus Creator3/9  "sp_PQ"
  sp_E [pu]/1 -> Bus Creator3/10  "sp_E"

== system AC_base_1_VSM_2_22a/Variant Subsystem3/VSM/Inverter AverageMdl LC SimScape2/Modul F30 fixed DC voltage Average SimScape/measMerge3/measMerge123 ==
  note: In Triphase Modell: Mittelwert aus allen dc Spannungen.
      | Da im Modell die DC Spannung identisch ist, wird die erste übergeben
  meas1 : Inport
  meas2 : Inport  Port=2
  meas3 : Inport  Port=3
  Bus Creator : BusCreator  Inputs=3
  Bus Creator2 : BusCreator  Inputs=8
  Bus Selector : BusSelector  OutputSignals=meas1.meas_u_cap,meas2.meas_u_cap,meas3.meas_u_cap
  Bus Selector1 : BusSelector  OutputSignals=meas1.meas_u_out,meas2.meas_u_out,meas3.meas_u_out
  Bus Selector2 : BusSelector  OutputSignals=meas1.meas_i_inverter,meas2.meas_i_inverter,meas3.meas_i_inverter
  Bus Selector3 : BusSelector  OutputSignals=meas1.meas_i_out,meas2.meas_i_out,meas3.meas_i_out
  Bus Selector4 : BusSelector  OutputSignals=meas1.connection_state  OutputAsBus=on
  Bus Selector5 : BusSelector  OutputSignals=meas1.enabled  OutputAsBus=on
  Bus Selector6 : BusSelector  OutputSignals=meas1.meas_u_dc  OutputAsBus=on
  Bus Selector7 : BusSelector  OutputSignals=meas1.block,meas3.block,meas2.block
  Bus to Vector4 : BusToVector  Commented=on
  Mux{,1..4} (5 alike) : Mux  Inputs=3
  meas : Outport  VectorParamsAs1DForOutWhenUnconnected=off
  wires:
  meas3/1 -> Bus Creator/3  "meas3"
  Bus Selector4/1 -> Bus Creator2/6  "connection_state"
  Bus Creator2/1 -> meas/1
  Mux3/1 -> Bus Creator2/5  "meas_i_out"
  Mux2/1 -> Bus Creator2/4  "meas_i_inverter"
  Mux1/1 -> Bus Creator2/3  "meas_u_out"
  Mux/1 -> Bus Creator2/2  "meas_u_cap"
  meas1/1 -> Bus Creator/1  "meas1"
  meas2/1 -> Bus Creator/2  "meas2"
  Bus Creator/1 -> Bus Selector7/1, Bus Selector5/1, Bus Selector4/1, Bus Selector3/1, Bus Selector2/1, Bus Selector1/1, Bus Selector/1, Bus Selector6/1
  Bus Selector5/1 -> Bus Creator2/7  "enabled"
  Bus Selector6/1 -> Bus Creator2/1  "meas_u_dc"
  Bus Selector/1 -> Mux/1  "<meas_u_cap>"
  Bus Selector/2 -> Mux/2  "<meas_u_cap>"
  Bus Selector/3 -> Mux/3  "<meas_u_cap>"
  Bus Selector1/1 -> Mux1/1  "<meas_u_out>"
  Bus Selector1/2 -> Mux1/2  "<meas_u_out>"
  Bus Selector1/3 -> Mux1/3  "<meas_u_out>"
  Bus Selector2/1 -> Mux2/1  "<meas_i_inverter>"
  Bus Selector2/2 -> Mux2/2  "<meas_i_inverter>"
  Bus Selector2/3 -> Mux2/3  "<meas_i_inverter>"
  Bus Selector3/1 -> Mux3/1  "<meas_i_out>"
  Bus Selector3/2 -> Mux3/2  "<meas_i_out>"
  Bus Selector3/3 -> Mux3/3  "<meas_i_out>"
  Bus Selector7/2 -> Mux4/2  "<block>"
  Bus Selector7/1 -> Mux4/1  "<block>"
  Bus Selector7/3 -> Mux4/3  "<block>"
  Mux4/1 -> Bus Creator2/8  "block"

== system AC_base_1_VSM_2_22a/Variant Subsystem3/VSM/Inverter AverageMdl LC SimScape2/Modul F30 fixed DC voltage Average SimScape/simscape_bridgefilter_aca/PWM Blocking1 ==
  i_inverter : Inport
  enable : Inport  Port=2
  AND2 : Logic  IconShape=distinctive  AllPortsSameDT=off  OutDataTypeStr=boolean
  AND3 : Logic  IconShape=distinctive  AllPortsSameDT=off  OutDataTypeStr=boolean
  Abs2 : Abs  SaturateOnIntegerOverflow=off
  Compare To Constant1 : simulink/Logic and Bit Operations/Compare To Constant  relop=<=  const=Ipwm_back  OutDataTypeStr=boolean
  Compare To Constant4 : simulink/Logic and Bit Operations/Compare To Constant  relop=>  const=Ipwm_off  OutDataTypeStr=boolean
  Data Type Conversion2 : DataTypeConversion  SaturateOnIntegerOverflow=off  RndMeth=Floor
  S-R Flip-Flop1 : simulink_extras/Flip Flops/S-R Flip-Flop  initial_condition=0
  Terminator1 : Terminator
  Trigger Spike at new Control Sample : Subsystem
  Unit Delay2 : UnitDelay  SampleTime=-1  HasFrameUpgradeWarning=on
  enable_blk : Outport
  wires:
  Trigger Spike at new Control Sample/1(y) -> AND2/1
  Compare To Constant1/1 -> AND2/2  "S"
  Unit Delay2/1 -> Abs2/1
  Abs2/1 -> Compare To Constant4/1, Compare To Constant1/1
  AND2/1 -> S-R Flip-Flop1/1
  Compare To Constant4/1 -> S-R Flip-Flop1/2  "R"
  S-R Flip-Flop1/1 -> AND3/2  "ena"
  Data Type Conversion2/1 -> enable_blk/1
  enable/1 -> AND3/1
  AND3/1 -> Data Type Conversion2/1
  S-R Flip-Flop1/2 -> Terminator1/1
  i_inverter/1 -> Unit Delay2/1

== system AC_base_1_VSM_2_22a/Variant Subsystem3/VSM/Inverter AverageMdl LC SimScape2/Modul F30 fixed DC voltage Average SimScape/simscape_bridgefilter_aca1/PWM Blocking1 ==
  i_inverter : Inport
  enable : Inport  Port=2
  AND2 : Logic  IconShape=distinctive  AllPortsSameDT=off  OutDataTypeStr=boolean
  AND3 : Logic  IconShape=distinctive  AllPortsSameDT=off  OutDataTypeStr=boolean
  Abs2 : Abs  SaturateOnIntegerOverflow=off
  Compare To Constant1 : simulink/Logic and Bit Operations/Compare To Constant  relop=<=  const=Ipwm_back  OutDataTypeStr=boolean
  Compare To Constant4 : simulink/Logic and Bit Operations/Compare To Constant  relop=>  const=Ipwm_off  OutDataTypeStr=boolean
  Data Type Conversion2 : DataTypeConversion  SaturateOnIntegerOverflow=off  RndMeth=Floor
  S-R Flip-Flop1 : simulink_extras/Flip Flops/S-R Flip-Flop  initial_condition=0
  Terminator1 : Terminator
  Trigger Spike at new Control Sample : Subsystem
  Unit Delay2 : UnitDelay  SampleTime=-1  HasFrameUpgradeWarning=on
  enable_blk : Outport
  wires:
  i_inverter/1 -> Unit Delay2/1
  S-R Flip-Flop1/2 -> Terminator1/1
  AND3/1 -> Data Type Conversion2/1
  enable/1 -> AND3/1
  Data Type Conversion2/1 -> enable_blk/1
  S-R Flip-Flop1/1 -> AND3/2  "ena"
  Compare To Constant4/1 -> S-R Flip-Flop1/2  "R"
  AND2/1 -> S-R Flip-Flop1/1
  Abs2/1 -> Compare To Constant1/1, Compare To Constant4/1
  Unit Delay2/1 -> Abs2/1
  Compare To Constant1/1 -> AND2/2  "S"
  Trigger Spike at new Control Sample/1(y) -> AND2/1

== system AC_base_1_VSM_2_22a/Variant Subsystem3/VSM/Inverter AverageMdl LC SimScape2/Modul F30 fixed DC voltage Average SimScape/simscape_bridgefilter_aca2/PWM Blocking1 ==
  i_inverter : Inport
  enable : Inport  Port=2
  AND2 : Logic  IconShape=distinctive  AllPortsSameDT=off  OutDataTypeStr=boolean
  AND3 : Logic  IconShape=distinctive  AllPortsSameDT=off  OutDataTypeStr=boolean
  Abs2 : Abs  SaturateOnIntegerOverflow=off
  Compare To Constant1 : simulink/Logic and Bit Operations/Compare To Constant  relop=<=  const=Ipwm_back  OutDataTypeStr=boolean
  Compare To Constant4 : simulink/Logic and Bit Operations/Compare To Constant  relop=>  const=Ipwm_off  OutDataTypeStr=boolean
  Data Type Conversion2 : DataTypeConversion  SaturateOnIntegerOverflow=off  RndMeth=Floor
  S-R Flip-Flop1 : simulink_extras/Flip Flops/S-R Flip-Flop  initial_condition=0
  Terminator1 : Terminator
  Trigger Spike at new Control Sample : Subsystem
  Unit Delay2 : UnitDelay  SampleTime=-1  HasFrameUpgradeWarning=on
  enable_blk : Outport
  wires:
  Trigger Spike at new Control Sample/1(y) -> AND2/1
  Compare To Constant1/1 -> AND2/2  "S"
  Unit Delay2/1 -> Abs2/1
  Abs2/1 -> Compare To Constant4/1, Compare To Constant1/1
  AND2/1 -> S-R Flip-Flop1/1
  Compare To Constant4/1 -> S-R Flip-Flop1/2  "R"
  S-R Flip-Flop1/1 -> AND3/2  "ena"
  Data Type Conversion2/1 -> enable_blk/1
  enable/1 -> AND3/1
  AND3/1 -> Data Type Conversion2/1
  S-R Flip-Flop1/2 -> Terminator1/1
  i_inverter/1 -> Unit Delay2/1

== system AC_base_1_VSM_2_22a/Variant Subsystem3/VSM/VSM1/VSM/CONTROL/Subsystem1 ==
  <R1> : Inport
  <L1> : Inport  Port=2
  I : Inport  Port=3
  U_i : Inport  Port=4
  Enable : EnablePort
  MATLAB Function : MATLAB Function  TreatAsAtomicUnit=on  SystemSampleTime=ControlSampleTime
  Selector : Selector  InputPortWidth=3  IndexOptions=Index vector (dialog)  Indices=[1 2]  OutputSizes=1
  Selector1 : Selector  InputPortWidth=3  IndexOptions=Index vector (dialog)  Indices=[1 2]  OutputSizes=1
  phi_vsm : Outport
  U_v : Outport  Port=2
  wires:
  MATLAB Function/2(U_v) -> U_v/1
  MATLAB Function/1(phi_vsm) -> phi_vsm/1
  U_i/1 -> Selector1/1
  I/1 -> Selector/1
  Selector1/1 -> MATLAB Function/4(U_i)
  Selector/1 -> MATLAB Function/1(I)
  <R1>/1 -> MATLAB Function/3(R1)
  <L1>/1 -> MATLAB Function/2(L1)
